simulink model "FluidDynamics"  (R2012b)
settings: Solver=ode45  StartTime=0.0  StopTime=10.0  RelTol=1e-3
undefined symbols (not defined in the file or in its folder): Aleak1, Aleak2, Aleak3, Aleak4, Aleak5, Aleakext, Aleakint, Ap, Be, Cd, P10, P20, Rho, V011, V021, Xlength, Xov, Xwidth
settings Model: Creator=HBALLEST  LastModifiedBy=HBALLEST

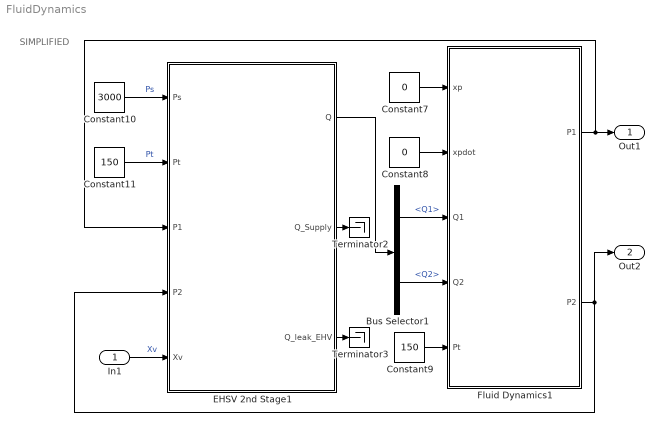
== system FluidDynamics ==
  note: SIMPLIFIED
  In1 : Inport
  Bus Selector1 : BusSelector  OutputSignals=Q1,Q2
  Constant10 : Constant  Value=3000
  Constant11 : Constant  Value=150
  Constant7 : Constant  Value=0
  Constant8 : Constant  Value=0
  Constant9 : Constant  Value=150
  EHSV 2nd Stage1 : Subsystem
  Fluid Dynamics1 : Subsystem
  Terminator2 : Terminator
  Terminator3 : Terminator
  Out1 : Outport
  Out2 : Outport  Port=2
  wires:
  Fluid Dynamics1/1(P1) -> EHSV 2nd Stage1/3(P1), Out1/1
  Fluid Dynamics1/2(P2) -> Out2/1, EHSV 2nd Stage1/4(P2)
  Constant7/1 -> Fluid Dynamics1/1(xp)
  Constant8/1 -> Fluid Dynamics1/2(xpdot)
  Constant9/1 -> Fluid Dynamics1/5(Pt)
  EHSV 2nd Stage1/1(Q) -> Bus Selector1/1
  Bus Selector1/1 -> Fluid Dynamics1/3(Q1)  "<Q1>"
  Bus Selector1/2 -> Fluid Dynamics1/4(Q2)  "<Q2>"
  EHSV 2nd Stage1/2(Q_Supply) -> Terminator2/1
  EHSV 2nd Stage1/3(Q_leak_EHV) -> Terminator3/1
  Constant11/1 -> EHSV 2nd Stage1/2(Pt)  "Pt"
  Constant10/1 -> EHSV 2nd Stage1/1(Ps)  "Ps"
  In1/1 -> EHSV 2nd Stage1/5(Xv)  "Xv"

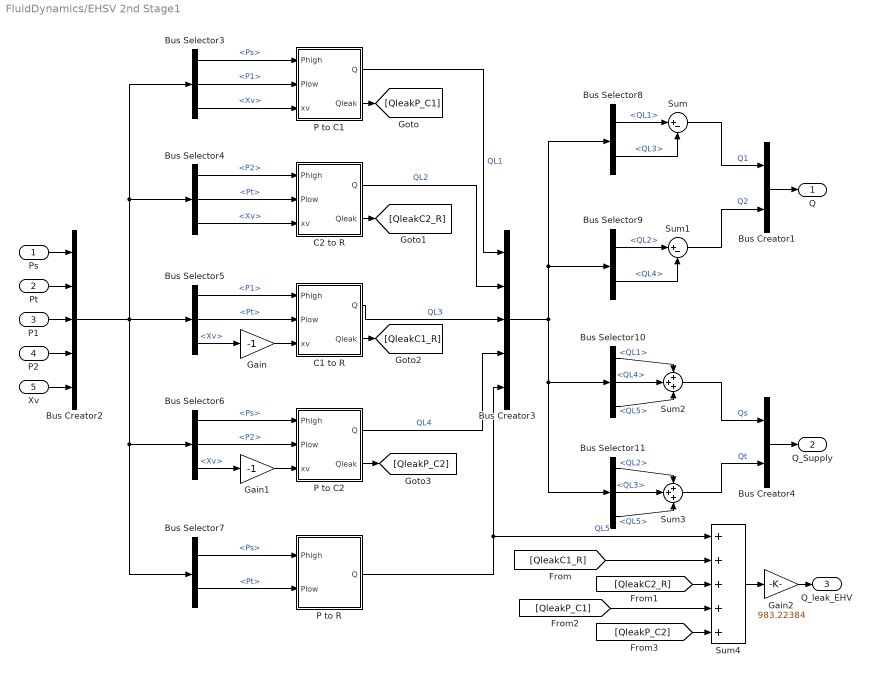
== system FluidDynamics/EHSV 2nd Stage1 ==
  Ps : Inport
  Pt : Inport  Port=2
  P1 : Inport  Port=3
  P2 : Inport  Port=4
  Xv : Inport  Port=5
  Bus Creator1 : BusCreator  Inputs=2
  Bus Creator2 : BusCreator  Inputs=5
  Bus Creator3 : BusCreator  Inputs=5
  Bus Creator4 : BusCreator  Inputs=2
  Bus Selector10 : BusSelector  OutputSignals=QL1,QL4,QL5
  Bus Selector11 : BusSelector  OutputSignals=QL2,QL3,QL5
  Bus Selector3 : BusSelector  OutputSignals=Ps,P1,Xv
  Bus Selector4 : BusSelector  OutputSignals=P2,Pt,Xv
  Bus Selector5 : BusSelector  OutputSignals=P1,Pt,Xv
  Bus Selector6 : BusSelector  OutputSignals=Ps,P2,Xv
  Bus Selector7 : BusSelector  OutputSignals=Ps,Pt
  Bus Selector8 : BusSelector  OutputSignals=QL1,QL3
  Bus Selector9 : BusSelector  OutputSignals=QL2,QL4
  C1 to R : Subsystem
  C2 to R : Subsystem
  Gain : Gain  Gain=-1
  Gain1 : Gain  Gain=-1
  Gain2 : Gain  Gain=983.22384
  P to C1 : Subsystem
  P to C2 : Subsystem
  P to R : Subsystem
  Sum : Sum  Inputs=|+-
  Sum1 : Sum  Inputs=|+-
  Sum2 : Sum  Inputs=+++
  Sum3 : Sum  Inputs=+++
  Sum4 : Sum  Inputs=+++++
  Q : Outport
  Q_Supply : Outport  Port=2
  Q_leak_EHV : Outport  Port=3
  wires:
  Bus Creator1/1 -> Q/1
  Bus Selector3/1 -> P to C1/1(Phigh)  "<Ps>"
  Bus Selector3/2 -> P to C1/2(Plow)  "<P1>"
  Bus Selector3/3 -> P to C1/3(xv)  "<Xv>"
  Bus Selector4/1 -> C2 to R/1(Phigh)  "<P2>"
  Bus Selector4/2 -> C2 to R/2(Plow)  "<Pt>"
  Bus Selector4/3 -> C2 to R/3(xv)  "<Xv>"
  Bus Selector5/3 -> Gain/1  "<Xv>"
  Bus Selector6/1 -> P to C2/1(Phigh)  "<Ps>"
  Bus Selector6/2 -> P to C2/2(Plow)  "<P2>"
  Bus Selector6/3 -> Gain1/1  "<Xv>"
  Bus Selector7/1 -> P to R/1(Phigh)  "<Ps>"
  Bus Selector7/2 -> P to R/2(Plow)  "<Pt>"
  Bus Selector5/1 -> C1 to R/1(Phigh)  "<P1>"
  Bus Selector5/2 -> C1 to R/2(Plow)  "<Pt>"
  P to C1/1(Q) -> Bus Creator3/1  "QL1"
  C2 to R/1(Q) -> Bus Creator3/2  "QL2"
  C1 to R/1(Q) -> Bus Creator3/3  "QL3"
  P to C2/1(Q) -> Bus Creator3/4  "QL4"
  P to R/1(Q) -> Sum4/1, Bus Creator3/5  "QL5"
  Bus Creator2/1 -> Bus Selector5/1, Bus Selector3/1, Bus Selector4/1, Bus Selector7/1, Bus Selector6/1
  Bus Selector8/1 -> Sum/1  "<QL1>"
  Bus Selector8/2 -> Sum/2  "<QL3>"
  Bus Selector9/1 -> Sum1/1  "<QL2>"
  Bus Selector9/2 -> Sum1/2  "<QL4>"
  Bus Selector10/1 -> Sum2/1  "<QL1>"
  Bus Selector10/2 -> Sum2/2  "<QL4>"
  Bus Selector10/3 -> Sum2/3  "<QL5>"
  Bus Selector11/1 -> Sum3/1  "<QL2>"
  Bus Selector11/2 -> Sum3/2  "<QL3>"
  Bus Selector11/3 -> Sum3/3  "<QL5>"
  Bus Creator4/1 -> Q_Supply/1
  Bus Creator3/1 -> Bus Selector8/1, Bus Selector9/1, Bus Selector11/1, Bus Selector10/1
  Sum/1 -> Bus Creator1/1  "Q1"
  Sum1/1 -> Bus Creator1/2  "Q2"
  Sum2/1 -> Bus Creator4/1  "Qs"
  Sum3/1 -> Bus Creator4/2  "Qt"
  Ps/1 -> Bus Creator2/1
  Pt/1 -> Bus Creator2/2
  P1/1 -> Bus Creator2/3
  P2/1 -> Bus Creator2/4
  Xv/1 -> Bus Creator2/5
  Gain/1 -> C1 to R/3(xv)
  Gain1/1 -> P to C2/3(xv)
  Sum4/1 -> Gain2/1
  P to C1/2(Qleak) -> [QleakP_C1]
  C2 to R/2(Qleak) -> [QleakC2_R]
  C1 to R/2(Qleak) -> [QleakC1_R]
  P to C2/2(Qleak) -> [QleakP_C2]
  [QleakC1_R] -> Sum4/2
  [QleakC2_R] -> Sum4/3
  [QleakP_C2] -> Sum4/5
  [QleakP_C1] -> Sum4/4
  Gain2/1 -> Q_leak_EHV/1

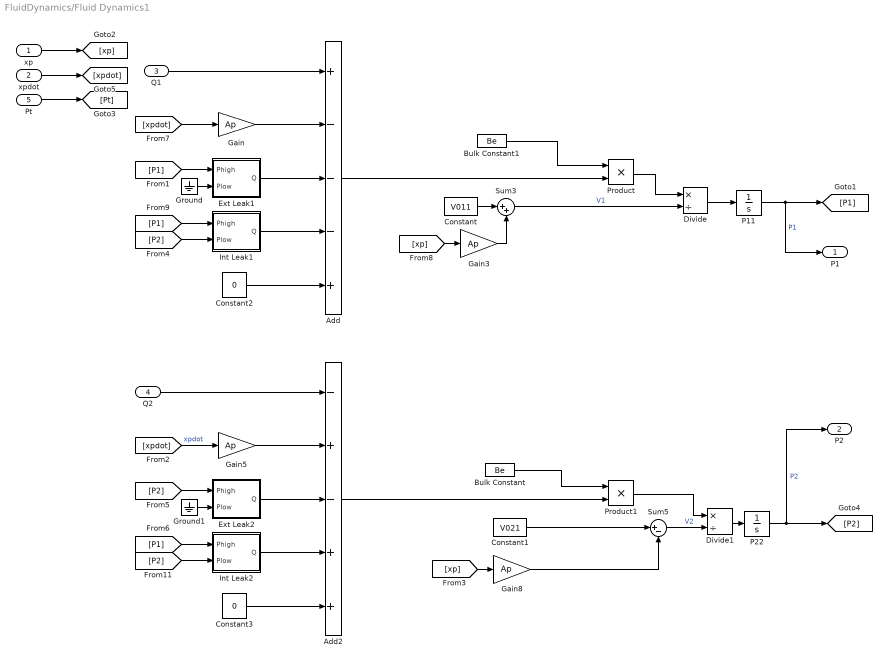
== system FluidDynamics/Fluid Dynamics1 ==
  xp : Inport
  xpdot : Inport  Port=2
  Q1 : Inport  Port=3
  Q2 : Inport  Port=4
  Pt : Inport  Port=5
  Add : Sum  Inputs=+---+
  Add2 : Sum  Inputs=-+-++
  Bulk Constant : Constant  Value=Be
  Bulk Constant1 : Constant  Value=Be
  Constant : Constant  Value=V011
  Constant1 : Constant  Value=V021
  Constant2 : Constant  Value=0
  Constant3 : Constant  Value=0
  Divide : Product  Inputs=*/
  Divide1 : Product  Inputs=*/
  Ext Leak1 : Subsystem
  Ext Leak2 : Subsystem
  Gain{,3,5,8} (4 alike) : Gain  Gain=Ap
  Ground : Ground
  Ground1 : Ground
  Int Leak1 : Subsystem
  Int Leak2 : Subsystem
  P11 : Integrator  InitialCondition=P10
  P22 : Integrator  InitialCondition=P20
  Product : Product  RndMeth=Zero
  Product1 : Product  RndMeth=Zero
  Sum3 : Sum  Inputs=|++
  Sum5 : Sum  Inputs=|+-
  P1 : Outport
  P2 : Outport  Port=2
  wires:
  Q1/1 -> Add/1
  [xpdot] -> Gain5/1  "xpdot"
  [xp] -> Gain8/1
  Int Leak2/1(Q) -> Add2/4
  Divide1/1 -> P22/1
  Sum5/1 -> Divide1/2  "V2"
  Gain8/1 -> Sum5/2
  Constant1/1 -> Sum5/1
  P22/1 -> [P2], P2/1  "P2"
  Ext Leak2/1(Q) -> Add2/3
  Gain5/1 -> Add2/2
  Int Leak1/1(Q) -> Add/4
  Divide/1 -> P11/1
  Sum3/1 -> Divide/2  "V1"
  Gain3/1 -> Sum3/2
  Constant/1 -> Sum3/1
  P11/1 -> P1/1, [P1]  "P1"
  Ext Leak1/1(Q) -> Add/3
  Add/1 -> Product/2
  Gain/1 -> Add/2
  [P1] -> Ext Leak1/1(Phigh)
  [P2] -> Ext Leak2/1(Phigh)
  xpdot/1 -> [xpdot]
  [xpdot] -> Gain/1
  xp/1 -> [xp]
  [xp] -> Gain3/1
  [P2] -> Int Leak1/2(Plow)
  Ground/1 -> Ext Leak1/2(Plow)
  Ground1/1 -> Ext Leak2/2(Plow)
  [P1] -> Int Leak2/1(Phigh)
  [P1] -> Int Leak1/1(Phigh)
  Constant2/1 -> Add/5
  [P2] -> Int Leak2/2(Plow)
  Constant3/1 -> Add2/5
  Pt/1 -> [Pt]
  Product/1 -> Divide/1
  Product1/1 -> Divide1/1
  Add2/1 -> Product1/2
  Bulk Constant/1 -> Product1/1
  Bulk Constant1/1 -> Product/1
  Q2/1 -> Add2/1

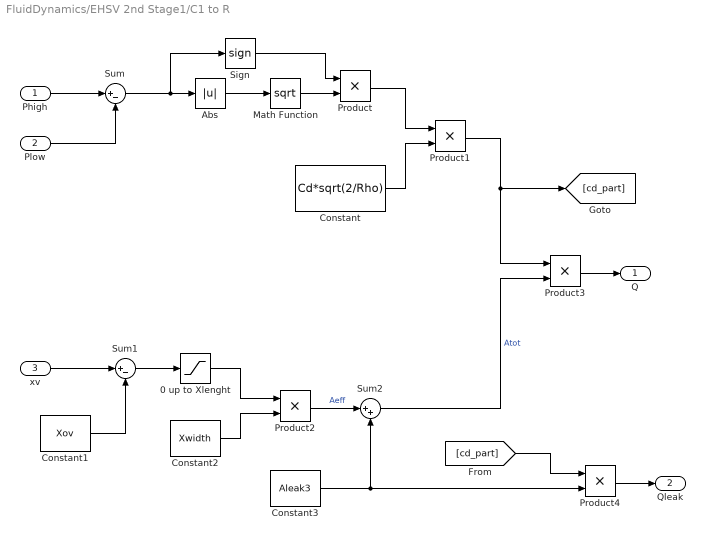
== system FluidDynamics/EHSV 2nd Stage1/C1 to R ==
  Phigh : Inport
  Plow : Inport  Port=2
  xv : Inport  Port=3
  0 up to Xlenght : Saturate  UpperLimit=Xlength  LowerLimit=0
  Abs : Abs
  Constant : Constant  Value=Cd*sqrt(2/Rho)
  Constant1 : Constant  Value=Xov
  Constant2 : Constant  Value=Xwidth
  Constant3 : Constant  Value=Aleak3
  Math Function : Math  Operator=sqrt  SaturateOnIntegerOverflow=on
  Product{,1..4} (5 alike) : Product  RndMeth=Zero
  Sign : Signum
  Sum : Sum  Inputs=|+-
  Sum1 : Sum  Inputs=|+-
  Sum2 : Sum  Inputs=|++
  Q : Outport
  Qleak : Outport  Port=2
  wires:
  Phigh/1 -> Sum/1
  Plow/1 -> Sum/2
  Sum/1 -> Abs/1, Sign/1
  Abs/1 -> Math Function/1
  Sign/1 -> Product/1
  Math Function/1 -> Product/2
  Constant/1 -> Product1/2
  Product/1 -> Product1/1
  xv/1 -> Sum1/1
  Constant1/1 -> Sum1/2
  Sum1/1 -> 0 up to Xlenght/1
  0 up to Xlenght/1 -> Product2/1
  Constant2/1 -> Product2/2
  Product2/1 -> Sum2/1  "Aeff"
  Constant3/1 -> Product4/2, Sum2/2
  Product1/1 -> [cd_part], Product3/1
  Sum2/1 -> Product3/2  "Atot"
  Product3/1 -> Q/1
  Product4/1 -> Qleak/1
  [cd_part] -> Product4/1

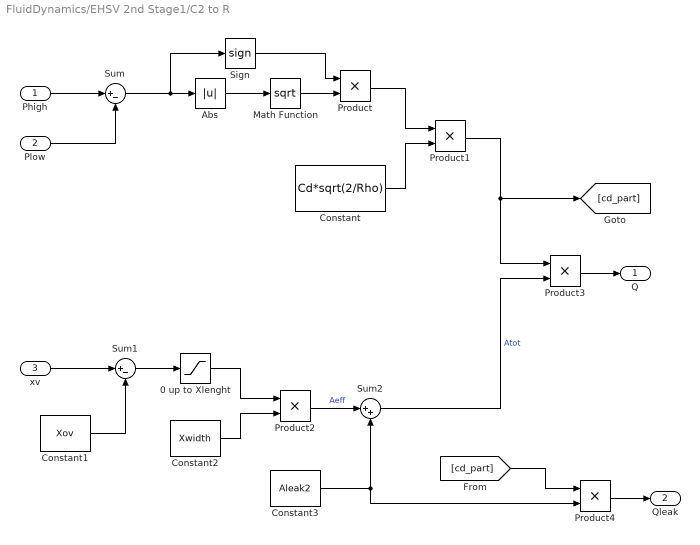
== system FluidDynamics/EHSV 2nd Stage1/C2 to R ==
  Phigh : Inport
  Plow : Inport  Port=2
  xv : Inport  Port=3
  0 up to Xlenght : Saturate  UpperLimit=Xlength  LowerLimit=0
  Abs : Abs
  Constant : Constant  Value=Cd*sqrt(2/Rho)
  Constant1 : Constant  Value=Xov
  Constant2 : Constant  Value=Xwidth
  Constant3 : Constant  Value=Aleak2
  Math Function : Math  Operator=sqrt  SaturateOnIntegerOverflow=on
  Product{,1..4} (5 alike) : Product  RndMeth=Zero
  Sign : Signum
  Sum : Sum  Inputs=|+-
  Sum1 : Sum  Inputs=|+-
  Sum2 : Sum  Inputs=|++
  Q : Outport
  Qleak : Outport  Port=2
  wires:
  Product3/1 -> Q/1
  Sum2/1 -> Product3/2  "Atot"
  Product1/1 -> [cd_part], Product3/1
  Product2/1 -> Sum2/1  "Aeff"
  Constant2/1 -> Product2/2
  0 up to Xlenght/1 -> Product2/1
  Sum1/1 -> 0 up to Xlenght/1
  Constant1/1 -> Sum1/2
  xv/1 -> Sum1/1
  Product/1 -> Product1/1
  Constant/1 -> Product1/2
  Math Function/1 -> Product/2
  Sign/1 -> Product/1
  Abs/1 -> Math Function/1
  Sum/1 -> Sign/1, Abs/1
  Plow/1 -> Sum/2
  Phigh/1 -> Sum/1
  Constant3/1 -> Product4/2, Sum2/2
  Product4/1 -> Qleak/1
  [cd_part] -> Product4/1

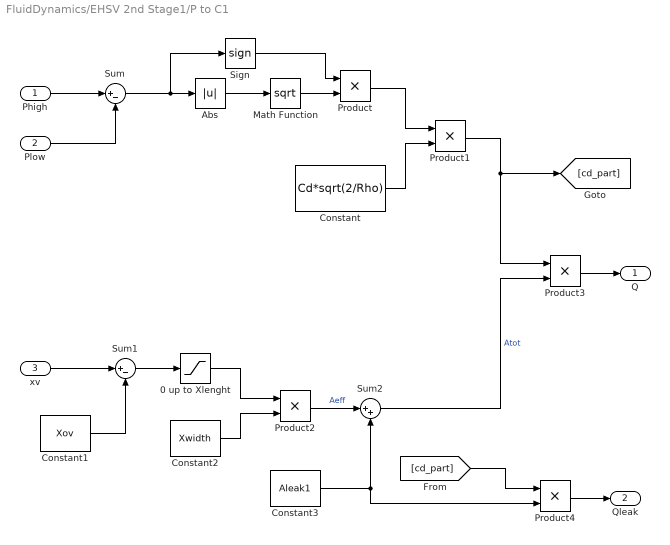
== system FluidDynamics/EHSV 2nd Stage1/P to C1 ==
  Phigh : Inport
  Plow : Inport  Port=2
  xv : Inport  Port=3
  0 up to Xlenght : Saturate  UpperLimit=Xlength  LowerLimit=0
  Abs : Abs
  Constant : Constant  Value=Cd*sqrt(2/Rho)
  Constant1 : Constant  Value=Xov
  Constant2 : Constant  Value=Xwidth
  Constant3 : Constant  Value=Aleak1
  Math Function : Math  Operator=sqrt  SaturateOnIntegerOverflow=on
  Product{,1..4} (5 alike) : Product  RndMeth=Zero
  Sign : Signum
  Sum : Sum  Inputs=|+-
  Sum1 : Sum  Inputs=|+-
  Sum2 : Sum  Inputs=|++
  Q : Outport
  Qleak : Outport  Port=2
  wires:
  Phigh/1 -> Sum/1
  Plow/1 -> Sum/2
  Sum/1 -> Abs/1, Sign/1
  Abs/1 -> Math Function/1
  Sign/1 -> Product/1
  Math Function/1 -> Product/2
  Constant/1 -> Product1/2
  Product/1 -> Product1/1
  xv/1 -> Sum1/1
  Constant1/1 -> Sum1/2
  Sum1/1 -> 0 up to Xlenght/1
  0 up to Xlenght/1 -> Product2/1
  Constant2/1 -> Product2/2
  Product2/1 -> Sum2/1  "Aeff"
  Constant3/1 -> Sum2/2, Product4/2
  Product1/1 -> [cd_part], Product3/1
  Sum2/1 -> Product3/2  "Atot"
  Product3/1 -> Q/1
  Product4/1 -> Qleak/1
  [cd_part] -> Product4/1

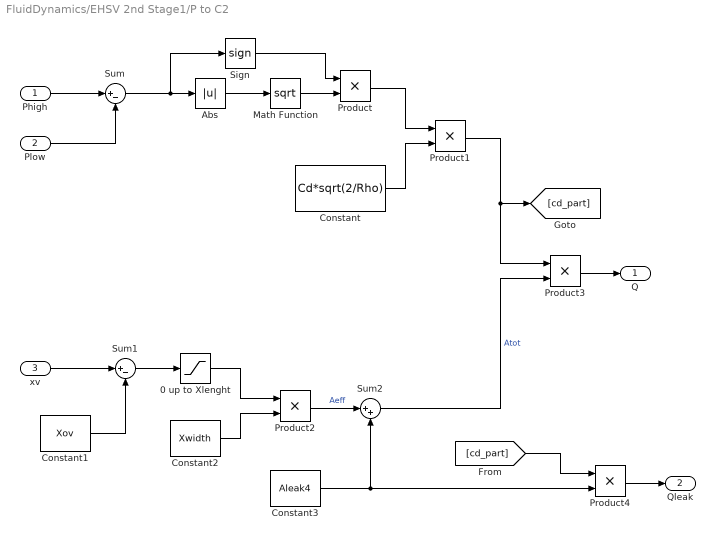
== system FluidDynamics/EHSV 2nd Stage1/P to C2 ==
  Phigh : Inport
  Plow : Inport  Port=2
  xv : Inport  Port=3
  0 up to Xlenght : Saturate  UpperLimit=Xlength  LowerLimit=0
  Abs : Abs
  Constant : Constant  Value=Cd*sqrt(2/Rho)
  Constant1 : Constant  Value=Xov
  Constant2 : Constant  Value=Xwidth
  Constant3 : Constant  Value=Aleak4
  Math Function : Math  Operator=sqrt  SaturateOnIntegerOverflow=on
  Product{,1..4} (5 alike) : Product  RndMeth=Zero
  Sign : Signum
  Sum : Sum  Inputs=|+-
  Sum1 : Sum  Inputs=|+-
  Sum2 : Sum  Inputs=|++
  Q : Outport
  Qleak : Outport  Port=2
  wires:
  Product3/1 -> Q/1
  Sum2/1 -> Product3/2  "Atot"
  Product1/1 -> [cd_part], Product3/1
  Product2/1 -> Sum2/1  "Aeff"
  Constant2/1 -> Product2/2
  0 up to Xlenght/1 -> Product2/1
  Sum1/1 -> 0 up to Xlenght/1
  Constant1/1 -> Sum1/2
  xv/1 -> Sum1/1
  Product/1 -> Product1/1
  Constant/1 -> Product1/2
  Math Function/1 -> Product/2
  Sign/1 -> Product/1
  Abs/1 -> Math Function/1
  Sum/1 -> Sign/1, Abs/1
  Plow/1 -> Sum/2
  Phigh/1 -> Sum/1
  Constant3/1 -> Sum2/2, Product4/2
  Product4/1 -> Qleak/1
  [cd_part] -> Product4/1

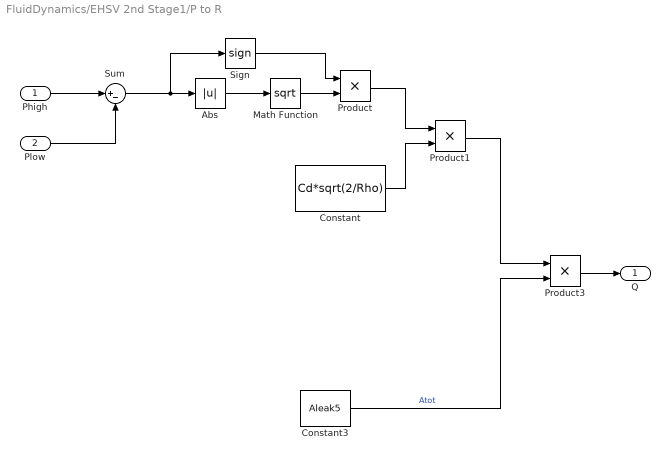
== system FluidDynamics/EHSV 2nd Stage1/P to R ==
  Phigh : Inport
  Plow : Inport  Port=2
  Abs : Abs
  Constant : Constant  Value=Cd*sqrt(2/Rho)
  Constant3 : Constant  Value=Aleak5
  Math Function : Math  Operator=sqrt  SaturateOnIntegerOverflow=on
  Product : Product  RndMeth=Zero
  Product1 : Product  RndMeth=Zero
  Product3 : Product  RndMeth=Zero
  Sign : Signum
  Sum : Sum  Inputs=|+-
  Q : Outport
  wires:
  Phigh/1 -> Sum/1
  Plow/1 -> Sum/2
  Sum/1 -> Abs/1, Sign/1
  Abs/1 -> Math Function/1
  Sign/1 -> Product/1
  Math Function/1 -> Product/2
  Constant/1 -> Product1/2
  Product/1 -> Product1/1
  Constant3/1 -> Product3/2  "Atot"
  Product1/1 -> Product3/1
  Product3/1 -> Q/1

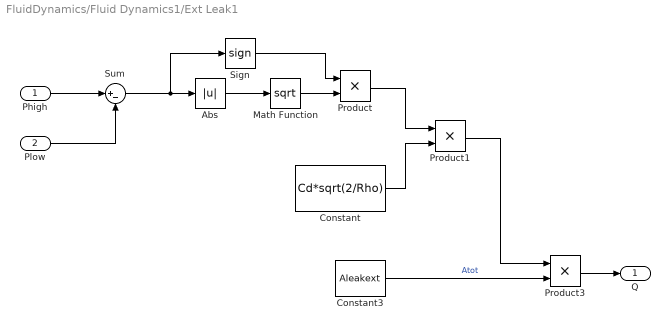
== system FluidDynamics/Fluid Dynamics1/Ext Leak1 ==
  Phigh : Inport
  Plow : Inport  Port=2
  Abs : Abs
  Constant : Constant  Value=Cd*sqrt(2/Rho)
  Constant3 : Constant  Value=Aleakext
  Math Function : Math  Operator=sqrt  SaturateOnIntegerOverflow=on
  Product : Product  RndMeth=Zero
  Product1 : Product  RndMeth=Zero
  Product3 : Product  RndMeth=Zero
  Sign : Signum
  Sum : Sum  Inputs=|+-
  Q : Outport
  wires:
  Phigh/1 -> Sum/1
  Sum/1 -> Abs/1, Sign/1
  Abs/1 -> Math Function/1
  Sign/1 -> Product/1
  Math Function/1 -> Product/2
  Constant/1 -> Product1/2
  Product/1 -> Product1/1
  Constant3/1 -> Product3/2  "Atot"
  Product1/1 -> Product3/1
  Product3/1 -> Q/1
  Plow/1 -> Sum/2

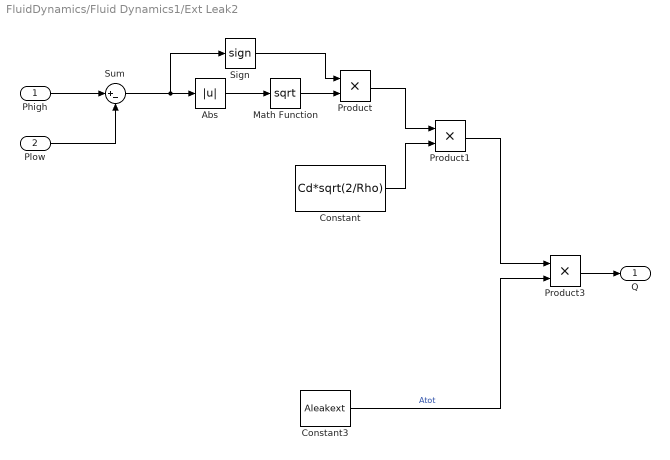
== system FluidDynamics/Fluid Dynamics1/Ext Leak2 ==
  Phigh : Inport
  Plow : Inport  Port=2
  Abs : Abs
  Constant : Constant  Value=Cd*sqrt(2/Rho)
  Constant3 : Constant  Value=Aleakext
  Math Function : Math  Operator=sqrt  SaturateOnIntegerOverflow=on
  Product : Product  RndMeth=Zero
  Product1 : Product  RndMeth=Zero
  Product3 : Product  RndMeth=Zero
  Sign : Signum
  Sum : Sum  Inputs=|+-
  Q : Outport
  wires:
  Plow/1 -> Sum/2
  Product3/1 -> Q/1
  Product1/1 -> Product3/1
  Constant3/1 -> Product3/2  "Atot"
  Product/1 -> Product1/1
  Constant/1 -> Product1/2
  Math Function/1 -> Product/2
  Sign/1 -> Product/1
  Abs/1 -> Math Function/1
  Sum/1 -> Sign/1, Abs/1
  Phigh/1 -> Sum/1

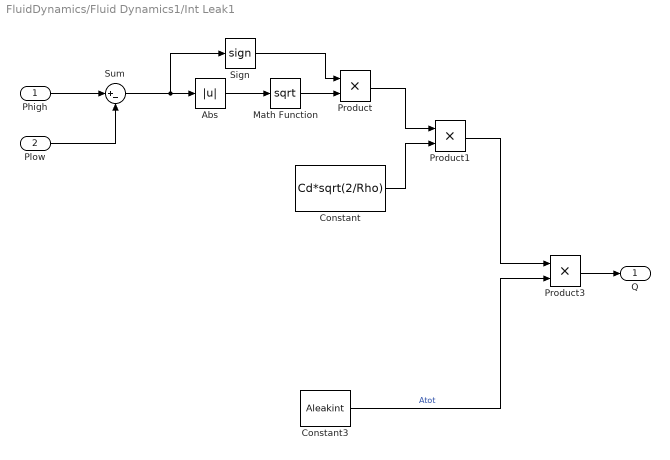
== system FluidDynamics/Fluid Dynamics1/Int Leak1 ==
  Phigh : Inport
  Plow : Inport  Port=2
  Abs : Abs
  Constant : Constant  Value=Cd*sqrt(2/Rho)
  Constant3 : Constant  Value=Aleakint
  Math Function : Math  Operator=sqrt  SaturateOnIntegerOverflow=on
  Product : Product  RndMeth=Zero
  Product1 : Product  RndMeth=Zero
  Product3 : Product  RndMeth=Zero
  Sign : Signum
  Sum : Sum  Inputs=|+-
  Q : Outport
  wires:
  Plow/1 -> Sum/2
  Product3/1 -> Q/1
  Product1/1 -> Product3/1
  Constant3/1 -> Product3/2  "Atot"
  Product/1 -> Product1/1
  Constant/1 -> Product1/2
  Math Function/1 -> Product/2
  Sign/1 -> Product/1
  Abs/1 -> Math Function/1
  Sum/1 -> Sign/1, Abs/1
  Phigh/1 -> Sum/1

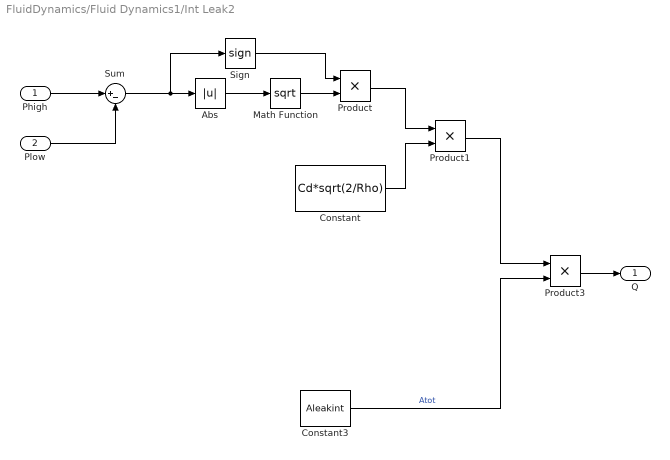
== system FluidDynamics/Fluid Dynamics1/Int Leak2 ==
  Phigh : Inport
  Plow : Inport  Port=2
  Abs : Abs
  Constant : Constant  Value=Cd*sqrt(2/Rho)
  Constant3 : Constant  Value=Aleakint
  Math Function : Math  Operator=sqrt  SaturateOnIntegerOverflow=on
  Product : Product  RndMeth=Zero
  Product1 : Product  RndMeth=Zero
  Product3 : Product  RndMeth=Zero
  Sign : Signum
  Sum : Sum  Inputs=|+-
  Q : Outport
  wires:
  Phigh/1 -> Sum/1
  Sum/1 -> Abs/1, Sign/1
  Abs/1 -> Math Function/1
  Sign/1 -> Product/1
  Math Function/1 -> Product/2
  Constant/1 -> Product1/2
  Product/1 -> Product1/1
  Constant3/1 -> Product3/2  "Atot"
  Product1/1 -> Product3/1
  Product3/1 -> Q/1
  Plow/1 -> Sum/2
